simulink library "csu_rdr_radar_lib_a"  (R2014b)
settings: Solver=ode45  SolverMode=SingleTasking  StartTime=0.0  StopTime=10.0  RelTol=1e-3
values from neighbouring files (symbols this model uses):
  rdr_position_in_lander = [radar_x radar_y radar_z]    [csu_rdr_radar_prep_a.m]
  rdr_rate_counter = rdr_update_time * 400    [csu_rdr_radar_prep_a.m]
undefined symbols (not defined in the file or in its folder): cam_cam1_lander_dcm, cam_image_plane_norm, ini_alt_wrt_1738rad, ini_tgt_landing_mcmf_pos, radar_position, rdr_bin_maximum, rdr_bin_minimum, rdr_null_meas, rdr_percent_error, rdr_range_max, rdr_range_min, sim_time_step_size
libraries: util_quat_lib x10, simulink x6, util_frame_rotation_lib x3, util_common_lib x2, util_info_lib x1, rotate_lib x1
settings Model: Creator=eleanor  LastModifiedBy=mstewart

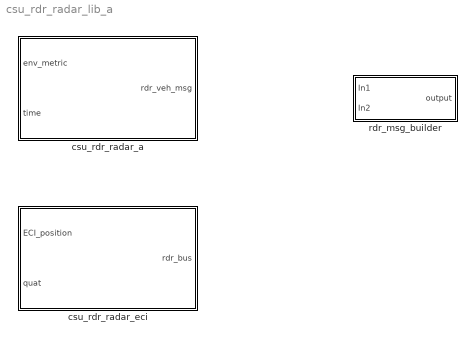
== system csu_rdr_radar_lib_a ==
  csu_rdr_radar_a : Subsystem  SystemSampleTime=0.1
  csu_rdr_radar_eci : Subsystem  SystemSampleTime=0.1
  rdr_msg_builder : Subsystem

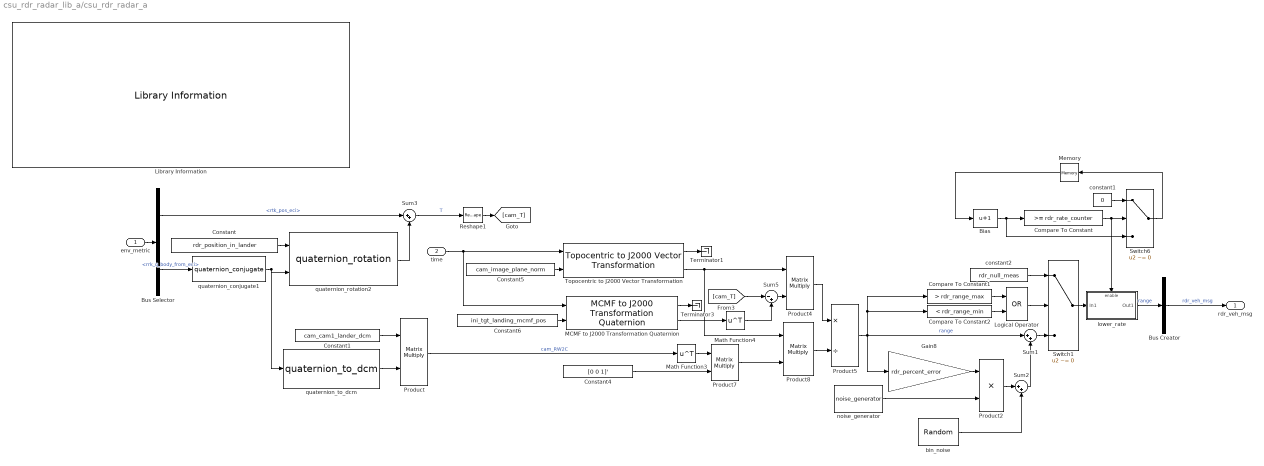
== system csu_rdr_radar_lib_a/csu_rdr_radar_a ==
  env_metric : Inport
  time : Inport  Port=2
  Bias : Bias  Bias=1
  Bus Creator : BusCreator  Inputs=1  OutDataTypeStr=Bus: rdr_veh_msg  NonVirtualBus=on
  Bus Selector : BusSelector  OutputSignals=lander_state_bus.rtk_pos_eci,lander_state_bus.rrk_q_body_from_eci
  Compare To Constant : simulink/Logic and Bit Operations/Compare To Constant  relop=>=  const=rdr_rate_counter  OutDataTypeStr=uint8
  Compare To Constant1 : simulink/Logic and Bit Operations/Compare To Constant  relop=>  const=rdr_range_max  OutDataTypeStr=uint8
  Compare To Constant2 : simulink/Logic and Bit Operations/Compare To Constant  relop=<  const=rdr_range_min  OutDataTypeStr=uint8
  Constant : Constant  Value=rdr_position_in_lander
  Constant1 : Constant  Value=cam_cam1_lander_dcm
  Constant4 : Constant  Value=[0 0 1]'  VectorParams1D=off
  Constant5 : Constant  Value=cam_image_plane_norm  VectorParams1D=off
  Constant6 : Constant  Value=ini_tgt_landing_mcmf_pos  VectorParams1D=off
  Gain8 : Gain  Gain=rdr_percent_error
  Library Information : util_info_lib/Library Information  owner='NONE'
  Logical Operator : Logic  Operator=OR  AllPortsSameDT=off  OutDataTypeStr=boolean
  MCMF to J2000 Transformation Quaternion : util_frame_rotation_lib/MCMF to J2000  Transformation Quaternion
  Math Function3 : Math  Operator=transpose  SaturateOnIntegerOverflow=on
  Math Function4 : Math  Operator=transpose  SaturateOnIntegerOverflow=on
  Memory : Memory  X0=rdr_rate_counter-1  InheritSampleTime=on
  Product{,4,7..8} (4 alike) : Product  Multiplication=Matrix(*)  RndMeth=Zero
  Product2 : Product  RndMeth=Zero
  Product5 : Product  Inputs=*/  RndMeth=Zero
  Reshape1 : Reshape  OutputDimensionality=Column vector (2-D)
  Sum1 : Sum  Inputs=|++
  Sum2 : Sum  Inputs=|++
  Sum3 : Sum  Inputs=|++
  Sum5 : Sum  Inputs=|-+
  Switch1 : Switch  Criteria=u2 ~= 0
  Switch6 : Switch  Criteria=u2 ~= 0  InputSameDT=on
  Terminator1 : Terminator
  Terminator3 : Terminator
  "Topocentric to J2000 Vector Transformation " : util_frame_rotation_lib/Topocentric to J2000 Vector Transformation   SystemSampleTime=-1
  bin_noise : UniformRandomNumber  Minimum=rdr_bin_minimum  Maximum=rdr_bin_maximum  SampleTime=sim_time_step_size
  constant1 : Constant  Value=0
  constant2 : Constant  Value=rdr_null_meas
  lower_rate : Subsystem  TreatAsAtomicUnit=on
  noise_generator : util_common_lib/noise_generator  std_dev=1  bias=0  seed=1  on=1  sample_time=sim_time_step_size
  quaternion_conjugate1 : util_quat_lib/quaternion_conjugate  SystemSampleTime=-1
  quaternion_rotation2 : util_quat_lib/quaternion_rotation  SystemSampleTime=-1
  quaternion_to_dcm : util_quat_lib/quaternion_to_dcm  SystemSampleTime=-1
  rdr_veh_msg : Outport
  wires:
  Constant4/1 -> Product7/2
  "Topocentric to J2000 Vector Transformation "/1 -> Terminator1/1
  "Topocentric to J2000 Vector Transformation "/2 -> Product8/1, Product4/1
  time/1 -> MCMF to J2000 Transformation Quaternion/1, "Topocentric to J2000 Vector Transformation "/1
  Constant6/1 -> MCMF to J2000 Transformation Quaternion/2
  Constant5/1 -> "Topocentric to J2000 Vector Transformation "/2
  Constant/1 -> quaternion_rotation2/1
  quaternion_rotation2/1 -> Sum3/2
  Constant1/1 -> Product/1
  quaternion_to_dcm/1 -> Product/2
  quaternion_conjugate1/1 -> quaternion_to_dcm/1, quaternion_rotation2/2
  Math Function4/1 -> Sum5/2
  MCMF to J2000 Transformation Quaternion/1 -> Terminator3/1
  MCMF to J2000 Transformation Quaternion/2 -> Math Function4/1
  Sum5/1 -> Product4/2
  [cam_T] -> Sum5/1
  Math Function3/1 -> Product7/1
  Reshape1/1 -> [cam_T]
  Product5/1 -> Gain8/1, Compare To Constant2/1, Compare To Constant1/1, Sum1/1  "range"
  Product7/1 -> Product8/2
  env_metric/1 -> Bus Selector/1
  Bus Selector/1 -> Sum3/1  "<rtk_pos_eci>"
  Bus Selector/2 -> quaternion_conjugate1/1  "<rrk_q_body_from_eci>"
  Product/1 -> Math Function3/1  "cam_RW2C"
  Sum3/1 -> Reshape1/1  "T"
  Product4/1 -> Product5/1
  Product8/1 -> Product5/2
  Memory/1 -> Bias/1
  Switch6/1 -> Memory/1
  Compare To Constant/1 -> lower_rate/Enable, Switch6/2
  Bias/1 -> Switch6/3, Compare To Constant/1
  constant1/1 -> Switch6/1
  lower_rate/1(Out1) -> Bus Creator/1  "range"
  Gain8/1 -> Product2/1
  noise_generator/1 -> Product2/2
  Bus Creator/1 -> rdr_veh_msg/1  "rdr_veh_msg"
  Product2/1 -> Sum2/1
  bin_noise/1 -> Sum2/2
  Compare To Constant1/1 -> Logical Operator/1
  Compare To Constant2/1 -> Logical Operator/2
  Logical Operator/1 -> Switch1/2
  Sum1/1 -> Switch1/3
  Sum2/1 -> Sum1/2
  constant2/1 -> Switch1/1
  Switch1/1 -> lower_rate/1(In1)

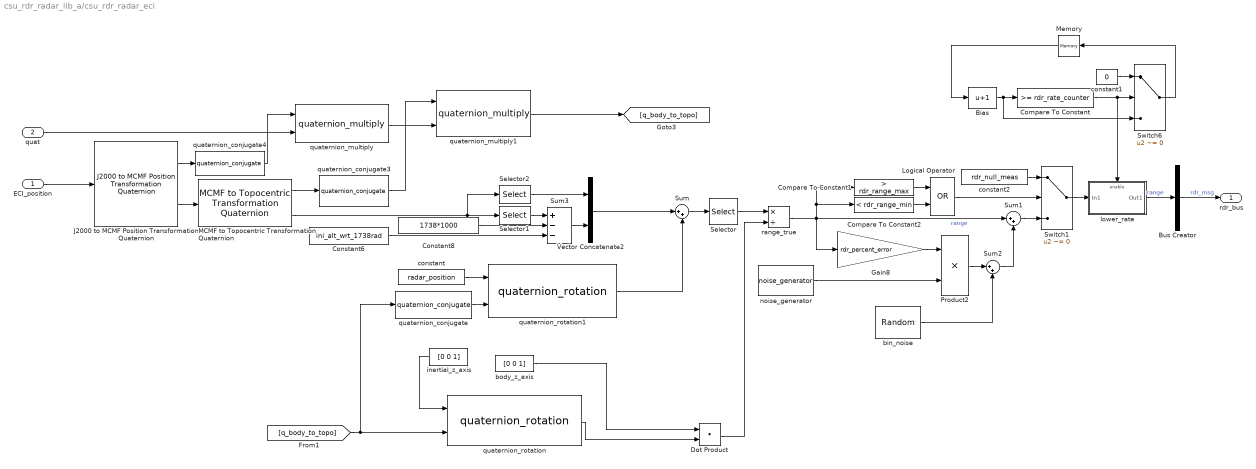
== system csu_rdr_radar_lib_a/csu_rdr_radar_eci ==
  ECI_position : Inport
  quat : Inport  Port=2
  Bias : Bias  Bias=1
  Bus Creator : BusCreator  Inputs=1
  Compare To Constant : simulink/Logic and Bit Operations/Compare To Constant  relop=>=  const=rdr_rate_counter  OutDataTypeStr=uint8
  Compare To Constant1 : simulink/Logic and Bit Operations/Compare To Constant  relop=>  const=rdr_range_max  OutDataTypeStr=uint8
  Compare To Constant2 : simulink/Logic and Bit Operations/Compare To Constant  relop=<  const=rdr_range_min  OutDataTypeStr=uint8
  Constant6 : Constant  Value=ini_alt_wrt_1738rad
  Constant8 : Constant  Value=1738*1000
  Dot Product : DotProduct  InputSameDT=on  OutDataTypeStr=Inherit: Inherit via internal rule
  Gain8 : Gain  Gain=rdr_percent_error
  J2000 to MCMF Position Transformation Quaternion : rotate_lib/J2000 to MCMF Position Transformation Quaternion
  Logical Operator : Logic  Operator=OR  AllPortsSameDT=off  OutDataTypeStr=boolean
  MCMF to Topocentric Transformation Quaternion : util_frame_rotation_lib/MCMF to Topocentric  Transformation Quaternion  SystemSampleTime=-1
  Memory : Memory  X0=rdr_rate_counter-1
  Product2 : Product  RndMeth=Zero
  Selector : Selector  InputPortWidth=3  Indices=[3]
  Selector1 : Selector  InputPortWidth=3  Indices=[3]
  Selector2 : Selector  InputPortWidth=3  Indices=[1 2]
  Sum : Sum  Inputs=|++
  Sum1 : Sum  Inputs=|++
  Sum2 : Sum  Inputs=|++
  Sum3 : Sum  Inputs=+--
  Switch1 : Switch  Criteria=u2 ~= 0
  Switch6 : Switch  Criteria=u2 ~= 0
  Vector Concatenate2 : Concatenate
  bin_noise : UniformRandomNumber  Minimum=rdr_bin_minimum  Maximum=rdr_bin_maximum  SampleTime=sim_time_step_size
  body_z_axis : Constant  Value=[0 0 1]
  constant : Constant  Value=radar_position
  constant1 : Constant  Value=0
  constant2 : Constant  Value=rdr_null_meas
  inertial_z_axis : Constant  Value=[0 0 1]
  lower_rate : Subsystem  TreatAsAtomicUnit=on
  noise_generator : util_common_lib/noise_generator  std_dev=1  bias=0  seed=1  on=1  sample_time=sim_time_step_size
  quaternion_conjugate : util_quat_lib/quaternion_conjugate  SystemSampleTime=-1
  quaternion_conjugate3 : util_quat_lib/quaternion_conjugate  SystemSampleTime=-1
  quaternion_conjugate4 : util_quat_lib/quaternion_conjugate  SystemSampleTime=-1
  quaternion_multiply : util_quat_lib/quaternion_multiply  SystemSampleTime=-1
  quaternion_multiply1 : util_quat_lib/quaternion_multiply  SystemSampleTime=-1
  quaternion_rotation : util_quat_lib/quaternion_rotation  SystemSampleTime=-1
  quaternion_rotation1 : util_quat_lib/quaternion_rotation  SystemSampleTime=-1
  range_true : Product  Inputs=*/  RndMeth=Zero
  rdr_bus : Outport
  wires:
  Memory/1 -> Bias/1
  Switch6/1 -> Memory/1
  Compare To Constant/1 -> lower_rate/Enable, Switch6/2
  Bias/1 -> Switch6/3, Compare To Constant/1
  constant1/1 -> Switch6/1
  lower_rate/1(Out1) -> Bus Creator/1  "range"
  Gain8/1 -> Product2/1
  noise_generator/1 -> Product2/2
  Bus Creator/1 -> rdr_bus/1  "rdr_msg"
  Selector/1 -> range_true/1
  body_z_axis/1 -> Dot Product/1
  inertial_z_axis/1 -> quaternion_rotation/1
  range_true/1 -> Gain8/1, Compare To Constant2/1, Compare To Constant1/1, Sum1/1  "range"
  Dot Product/1 -> range_true/2
  quaternion_rotation/1 -> Dot Product/2
  Sum/1 -> Selector/1
  quaternion_conjugate/1 -> quaternion_rotation1/2
  quaternion_rotation1/1 -> Sum/2
  constant/1 -> quaternion_rotation1/1
  Product2/1 -> Sum2/1
  bin_noise/1 -> Sum2/2
  Compare To Constant1/1 -> Logical Operator/1
  Compare To Constant2/1 -> Logical Operator/2
  Logical Operator/1 -> Switch1/2
  Sum1/1 -> Switch1/3
  Sum2/1 -> Sum1/2
  constant2/1 -> Switch1/1
  Switch1/1 -> lower_rate/1(In1)
  ECI_position/1 -> J2000 to MCMF Position Transformation Quaternion/1
  J2000 to MCMF Position Transformation Quaternion/2 -> MCMF to Topocentric Transformation Quaternion/1
  MCMF to Topocentric Transformation Quaternion/2 -> Selector1/1, Selector2/1
  Constant6/1 -> Sum3/3
  Constant8/1 -> Sum3/2
  Selector2/1 -> Vector Concatenate2/1
  Selector1/1 -> Sum3/1
  Sum3/1 -> Vector Concatenate2/2
  Vector Concatenate2/1 -> Sum/1
  quaternion_multiply1/1 -> [q_body_to_topo]
  MCMF to Topocentric Transformation Quaternion/1 -> quaternion_conjugate3/1
  quaternion_conjugate3/1 -> quaternion_multiply1/1
  quaternion_multiply/1 -> quaternion_multiply1/2
  J2000 to MCMF Position Transformation Quaternion/1 -> quaternion_conjugate4/1
  quat/1 -> quaternion_multiply/2
  quaternion_conjugate4/1 -> quaternion_multiply/1
  [q_body_to_topo] -> quaternion_rotation/2, quaternion_conjugate/1

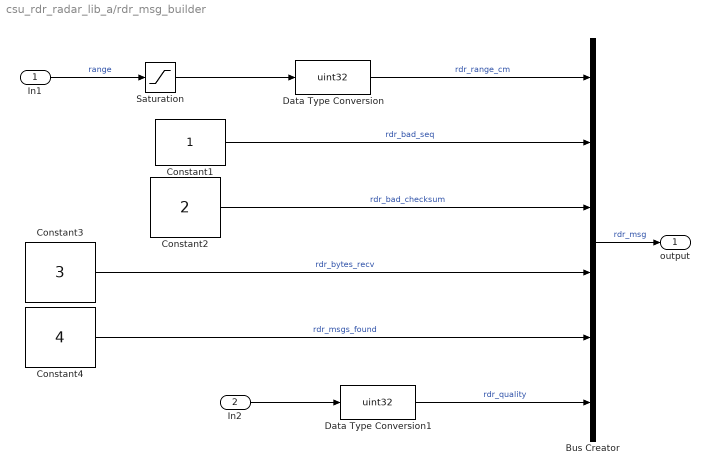
== system csu_rdr_radar_lib_a/rdr_msg_builder ==
  In1 : Inport
  In2 : Inport  Port=2
  Bus Creator : BusCreator  Inputs='rdr_range_cm','rdr_bad_seq','rdr_bad_checksum','rdr_bytes_recv','rdr_msgs_found','rdr_quality'
  Constant1 : Constant  OutDataTypeStr=uint32
  Constant2 : Constant  Value=2  OutDataTypeStr=uint32
  Constant3 : Constant  Value=3  OutDataTypeStr=uint32
  Constant4 : Constant  Value=4  OutDataTypeStr=uint32
  Data Type Conversion : DataTypeConversion  OutDataTypeStr=uint32  SaturateOnIntegerOverflow=on
  Data Type Conversion1 : DataTypeConversion  OutDataTypeStr=uint32  SaturateOnIntegerOverflow=on
  Saturation : Saturate  UpperLimit=4.2950e+009  LowerLimit=0
  output : Outport
  wires:
  In2/1 -> Data Type Conversion1/1
  Data Type Conversion1/1 -> Bus Creator/6  "rdr_quality"
  Constant4/1 -> Bus Creator/5  "rdr_msgs_found"
  Constant3/1 -> Bus Creator/4  "rdr_bytes_recv"
  Constant2/1 -> Bus Creator/3  "rdr_bad_checksum"
  Constant1/1 -> Bus Creator/2  "rdr_bad_seq"
  Bus Creator/1 -> output/1  "rdr_msg"
  Data Type Conversion/1 -> Bus Creator/1  "rdr_range_cm"
  In1/1 -> Saturation/1  "range"
  Saturation/1 -> Data Type Conversion/1

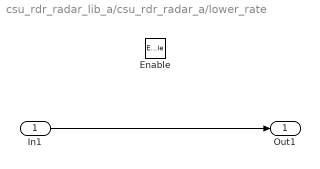
== system csu_rdr_radar_lib_a/csu_rdr_radar_a/lower_rate ==
  In1 : Inport
  Enable : EnablePort
  Out1 : Outport
  wires:
  In1/1 -> Out1/1

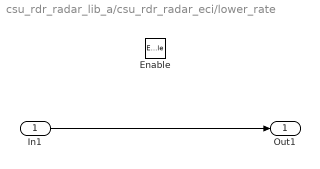
== system csu_rdr_radar_lib_a/csu_rdr_radar_eci/lower_rate ==
  In1 : Inport
  Enable : EnablePort
  Out1 : Outport
  wires:
  In1/1 -> Out1/1
